simulink model "all_sliding_mode_z_trajectory_extension_v1"  (R2016b)
settings: Solver=ode4  StartTime=0.0  StopTime=t_stop  FixedStep=t_step  MaxStep=0.00001  MinStep=0.00000000001  RelTol=1e-3  EnableMultiTasking=on
values from neighbouring files (symbols this model uses):
  g = single(9.81)    [covert_pressure_to_height.m]
undefined symbols (not defined in the file or in its folder): a1, a2, a3, a4, a5, a6, b, cm, ct, d, disturbance, fd, Ix, Ixx, Iy, Iyy, Iz, Izz, k1, k2, k3, k4, k5, k6, Kd_phi, Kd_theta, Kd_x, Kd_y, Kd_z, Ki_phi, Ki_theta, Ki_x, Ki_y, Ki_z, Kp_phi, Kp_theta, Kp_x, Kp_y, Kp_z, L, l1, l2, l3, l4, l5, l6, m, O, phi_init, phi_ref, psi_init, psi_ref, smc, tau_att, tau_att_1, tau_p, theta_init, theta_ref, xref, yref ... (+2)
libraries: simulink x2
settings Model: Creator=Ajinkya  LastModifiedBy=Ajinkya
settings SolverCC: ZeroCrossAlgorithm=Adaptive  AlgebraicLoopSolver=LineSearch
settings DataIOCC: LimitDataPoints=on  SaveFormat=StructureWithTime
settings OptimizationCC: DefaultParameterBehavior=Inlined  EfficientMapNaN2IntZero=off
settings DebuggingCC: ParameterOverflowMsg=warning  ParameterTunabilityLossMsg=error  SFUnexpectedBacktrackingDiag=warning  SFNoUnconditionalDefaultTransitionDiag=warning  SFExecutionAtInitializationDiag=none
settings HardwareCC: ProdBitPerSizeT=32  ProdBitPerPtrDiffT=32  ProdWordSize=32  ProdHWDeviceType=Specified  TargetBitPerPointer=64  TargetBitPerSizeT=64  TargetBitPerPtrDiffT=64  TargetLongLongMode=on  TargetIntDivRoundTo=Zero  TargetEndianess=LittleEndian  TargetWordSize=64  TargetHWDeviceType=MATLAB Host  ProdEqTarget=off
settings ModelReferenceCC: PropagateSignalLabelsOutOfModel=off
settings RTWCC: GenerateReport=on  LaunchReport=on
settings CodeAppCC: ForceParamTrailComments=on  MaxIdLength=128  OperatorAnnotations=on  MATLABSourceComments=on
settings GRTTargetCC: TargetLangStandard=C89/C90 (ANSI)
settings ConfigComp: CovMetricSettings=dw  CovHtmlReporting=on  CovSaveCumulativeToWorkspaceVar=on  CovSaveSingleToWorkspaceVar=on  CovExternalEMLEnable=off

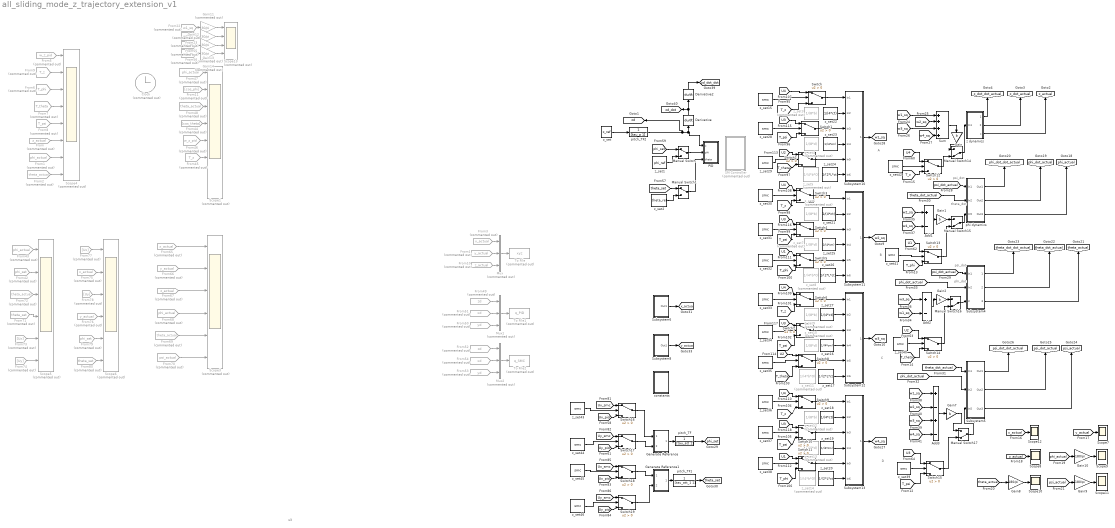
== system all_sliding_mode_z_trajectory_extension_v1 ==
  note: s3
  note: theta_dot
  note: psi_dot
  note: phi_dot
  note: psi_dot
  note: D
  note: C
  note: B
  note: A
  Add1 : Sum  Inputs=+-
  Add2 : Sum  Inputs=+-
  Add3 : Sum  Inputs=+-+-
  Clock : Clock  Commented=on
  Derivative : Derivative
  Derivative2 : Derivative
  From : From  Commented=on  GotoTag=z_actual  TagVisibility=global
  From{1,43,47,68} (4 alike) : From  Commented=on  GotoTag=phi_actual  TagVisibility=global
  From10 : From  Commented=on  GotoTag=z_actual  TagVisibility=global
  From11 : From  Commented=on  GotoTag=cos_phi
  From{2,48,69,72} (4 alike) : From  Commented=on  GotoTag=theta_actual  TagVisibility=global
  From22 : From  Commented=on  GotoTag=w1_sq  TagVisibility=global
  From23 : From  Commented=on  GotoTag=w2_sq  TagVisibility=global
  From3 : From  Commented=on  GotoTag=x_actual  TagVisibility=global
  From4 : From  Commented=on  GotoTag=y_actual  TagVisibility=global
  From42 : From  Commented=on  GotoTag=phi_set  TagVisibility=global
  From44 : From  Commented=on  GotoTag=cos_theta
  From45 : From  Commented=on  GotoTag=T_z  TagVisibility=global
  From46 : From  Commented=on  GotoTag=w_z_pid  TagVisibility=global
  From49 : From  Commented=on  GotoTag=zd  TagVisibility=global
  From5 : From  Commented=on  GotoTag=w_z_pid
  From50 : From  Commented=on  GotoTag=yd  TagVisibility=global
  From51 : From  Commented=on  GotoTag=xd  TagVisibility=global
  From52 : From  Commented=on  GotoTag=zd
  From53 : From  Commented=on  GotoTag=yd
  From54 : From  Commented=on  GotoTag=xd
  From55 : From  Commented=on  GotoTag=w3_sq  TagVisibility=global
  From56 : From  Commented=on  GotoTag=w4_sq  TagVisibility=global
  From6 : From  Commented=on  GotoTag=T_phi
  From65 : From  Commented=on  GotoTag=x_actual  TagVisibility=global
  From66 : From  Commented=on  GotoTag=y_actual  TagVisibility=global
  From67 : From  Commented=on  GotoTag=z_actual  TagVisibility=global
  From7 : From  Commented=on  GotoTag=T_theta
  From70 : From  Commented=on  GotoTag=psi_actual  TagVisibility=global
  From71 : From  Commented=on  GotoTag=theta_set  TagVisibility=global
  From73 : From  Commented=on  GotoTag=Ux
  From74 : From  Commented=on  GotoTag=Uy
  From75 : From  Commented=on  GotoTag=x_actual  TagVisibility=global
  From76 : From  Commented=on  GotoTag=y_actual  TagVisibility=global
  From77 : From  Commented=on  GotoTag=Ux
  From78 : From  Commented=on  GotoTag=Uy
  From79 : From  Commented=on  GotoTag=phi_set  TagVisibility=global
  From8 : From  Commented=on  GotoTag=T_psi
  From80 : From  Commented=on  GotoTag=theta_set  TagVisibility=global
  From9 : From  Commented=on  GotoTag=T_z
  Gain{,1..2,7} (4 alike) : Gain  Gain=b
  Gain10 : Gain  Gain=180/pi
  Gain{11..14} (4 alike) : Gain  Commented=on  Gain=30/pi
  Gain8 : Gain  Gain=180/pi
  Gain9 : Gain  Gain=180/pi
  Generate Reference : Subsystem
  Generate Reference1 : Subsystem
  Manual Switch : ManualSwitch
  Manual Switch1 : ManualSwitch
  Manual Switch{14..17} (4 alike) : ManualSwitch  CurrentSetting=0
  Mux : Mux  Commented=on  Inputs=3
  Mux1 : Mux  Commented=on  Inputs=3
  Mux2 : Mux  Commented=on  Inputs=3
  PID : Subsystem
  SM Controller : Subsystem  Commented=on
  Scope1 : Scope  Commented=on  NumInputPorts=8
  Scope{7..12} (6 alike) : Scope
  Scope13 : Scope  Commented=on  NumInputPorts=4
  Scope3 : Scope  Commented=on  NumInputPorts=6
  Scope4 : Scope  Commented=on  NumInputPorts=8
  Scope5 : Scope  Commented=on  NumInputPorts=6
  Scope6 : Scope  Commented=on  NumInputPorts=6
  Subsystem10 : Subsystem
  Subsystem11 : Subsystem
  Subsystem12 : Subsystem
  Subsystem13 : Subsystem
  Subsystem4 : Subsystem
  Subsystem5 : Subsystem
  Subsystem6 : Subsystem
  Subsystem8 : Subsystem
  Sum : Sum  Inputs=++++
  Switch{,1..19} (20 alike) : Switch  Criteria=u2 > Threshold
  To File : ToFile  Commented=on  Filename=xyz  MatrixName=xyz
  To File1 : ToFile  Commented=on  Filename=q_PID  MatrixName=q_PID
  To File2 : ToFile  Commented=on  Filename=q_SMC  MatrixName=q_SMC
  constants : Subsystem
  phi dynamics : Subsystem
  pitch_TF : TransferFcn  Denominator=[tau_att 1]
  pitch_TF1 : TransferFcn  Denominator=[tau_att_1 1]
  pitch_TF2 : TransferFcn  Denominator=[tau_p 1]
  z dynamics : Subsystem
  z_set : Constant  Value=z_ref
  z_set1 : Constant  Value=phi_ref
  z_set{4,7,10,13} (4 alike) : Constant  Commented=on  Value=1/(8*d)
  z_set{5,8,11,14} (4 alike) : Constant  Commented=on  Value=1/(4*b*O)
  z_set{3,6,9,12} (4 alike) : Constant  Commented=on  Value=1/(8*b)
  z_set{15,28..46} (20 alike) : Constant  Value=smc
  z_set{16,19,23,25} (4 alike) : Constant  Value=1/(4*cm)
  z_set{17,20,24,26} (4 alike) : Constant  Value=1/(2*L*ct)
  z_set{18,21..22,27} (4 alike) : Constant  Value=1/(4*ct)
  z_set2 : Constant  Value=theta_ref
  tag scope: phi_actual=global, phi_dot_actual=global, phi_dot_dot_actual=global, phi_set=global, psi_actual=global, psi_dot_actual=global, psi_dot_dot_actual=global, theta_actual=global, theta_dot_actual=global, theta_dot_dot_actual=global, theta_set=global, w1_sq=global, w2_sq=global, w3_sq=global, w4_sq=global, x_actual=global, y_actual=global, z_actual=global, z_dot_actual=global, z_dot_dot_actual=global, zd=global, zd_dot=global, zd_dot_dot=global
  wires:
  z_set/1 -> pitch_TF2/1
  z dynamics/1(z dot dot) -> [z_dot_dot_actual]
  z dynamics/2(z dot) -> [z_dot_actual]
  z dynamics/3(z) -> [z_actual]
  [w1_sq] -> Sum/1
  [w2_sq] -> Sum/2
  [w3_sq] -> Sum/3
  [w4_sq] -> Sum/4
  [psi_dot_actual] -> phi dynamics/1(In1)
  [theta_dot_actual] -> phi dynamics/2(In2)
  phi dynamics/1(Out1) -> [phi_dot_dot_actual]
  phi dynamics/2(Out2) -> [phi_dot_actual]
  phi dynamics/3(Out3) -> [phi_actual]
  [psi_dot_actual] -> Subsystem4/1(In1)
  [phi_dot_actual] -> Subsystem4/2(In2)
  Subsystem4/1(Out1) -> [theta_dot_dot_actual]
  Subsystem4/2(Out2) -> [theta_dot_actual]
  Subsystem4/3(Out3) -> [theta_actual]
  [theta_dot_actual] -> Subsystem5/1(In1)
  [phi_dot_actual] -> Subsystem5/2(In2)
  Subsystem5/1(Out1) -> [psi_dot_dot_actual]
  Subsystem5/2(Out2) -> [psi_dot_actual]
  Subsystem5/3(Out3) -> [psi_actual]
  From2/1 -> Scope4/8
  From1/1 -> Scope4/7
  From/1 -> Scope4/6
  From8/1 -> Scope4/5
  From7/1 -> Scope4/4
  From6/1 -> Scope4/3
  From9/1 -> Scope4/2
  From5/1 -> Scope4/1
  From11/1 -> Scope1/2
  From44/1 -> Scope1/4
  From45/1 -> Scope1/6
  From46/1 -> Scope1/5
  From48/1 -> Scope1/3
  From47/1 -> Scope1/1
  [w1_sq] -> Add2/2
  [w4_sq] -> Add3/4
  [w3_sq] -> Add3/3
  [w2_sq] -> Add3/2
  z_set1/1 -> Manual Switch/2
  [phi_set] -> Manual Switch/1
  z_set2/1 -> Manual Switch1/2
  [theta_set] -> Manual Switch1/1
  Subsystem6/1(Out1) -> [x_actual]
  Subsystem8/1(Out1) -> [y_actual]
  From65/1 -> Scope3/1
  From66/1 -> Scope3/2
  From67/1 -> Scope3/3
  From68/1 -> Scope3/4
  From69/1 -> Scope3/5
  From70/1 -> Scope3/6
  From42/1 -> Scope5/2
  From43/1 -> Scope5/1
  From71/1 -> Scope5/4
  From72/1 -> Scope5/3
  From73/1 -> Scope5/5
  From74/1 -> Scope5/6
  From75/1 -> Scope6/2
  From76/1 -> Scope6/4
  From77/1 -> Scope6/1
  From78/1 -> Scope6/3
  From79/1 -> Scope6/5
  From80/1 -> Scope6/6
  Derivative/1 -> [zd_dot], Derivative2/1
  Derivative2/1 -> [zd_dot_dot]
  Sum/1 -> Gain/1
  Manual Switch14/1 -> z dynamics/1(In1)
  Gain/1 -> Manual Switch14/1
  [w2_sq] -> Add1/1
  [w4_sq] -> Add1/2
  Manual Switch15/1 -> phi dynamics/3(In5)
  [w3_sq] -> Add2/1
  Manual Switch16/1 -> Subsystem4/3(w3_sq)
  Add1/1 -> Gain1/1
  Gain1/1 -> Manual Switch15/1
  Gain2/1 -> Manual Switch16/1
  Add2/1 -> Gain2/1
  [w1_sq] -> Add3/1
  Add3/1 -> Gain7/1
  Gain7/1 -> Manual Switch17/1
  Manual Switch17/1 -> Subsystem5/3(In5)
  z_set22/1 -> Subsystem10/2(In2)
  z_set23/1 -> Subsystem10/4(In4)
  z_set24/1 -> Subsystem10/6(In6)
  z_set21/1 -> Subsystem11/2(In2)
  z_set25/1 -> Subsystem11/4(In4)
  z_set26/1 -> Subsystem11/6(In6)
  z_set27/1 -> Subsystem12/2(In2)
  z_set16/1 -> Subsystem12/4(In4)
  z_set17/1 -> Subsystem12/6(In6)
  z_set18/1 -> Subsystem13/2(In2)
  z_set19/1 -> Subsystem13/4(In4)
  z_set20/1 -> Subsystem13/6(In6)
  Subsystem10/1(w1_sq) -> [w1_sq]
  Subsystem11/1(w2_sq) -> [w2_sq]
  Subsystem12/1(w3_sq) -> [w3_sq]
  Subsystem13/1(w4_sq) -> [w4_sq]
  [T_z] -> Switch/3
  Switch/1 -> Subsystem10/1(In1)
  [U4] -> Switch/1
  [T_z] -> Switch3/3
  [U4] -> Switch3/1
  Switch3/1 -> Subsystem11/1(In1)
  [T_z] -> Switch6/3
  Switch6/1 -> Subsystem12/1(In1)
  [U4] -> Switch6/1
  [T_z] -> Switch9/3
  Switch9/1 -> Subsystem13/1(In1)
  [U4] -> Switch9/1
  Switch1/1 -> Subsystem10/3(In3)
  [T_psi] -> Switch1/3
  Switch2/1 -> Subsystem10/5(In5)
  [T_theta] -> Switch2/3
  [T_psi] -> Switch4/3
  Switch4/1 -> Subsystem11/3(In3)
  Switch5/1 -> Subsystem11/5(In5)
  [T_phi] -> Switch5/3
  Switch7/1 -> Subsystem12/3(In3)
  [T_psi] -> Switch7/3
  Switch8/1 -> Subsystem12/5(In5)
  [T_theta] -> Switch8/3
  Switch10/1 -> Subsystem13/3(In3)
  [T_psi] -> Switch10/3
  Switch11/1 -> Subsystem13/5(In5)
  [T_phi] -> Switch11/3
  [U1] -> Switch5/1
  [U1] -> Switch11/1
  [U2] -> Switch2/1
  [U2] -> Switch8/1
  [U3] -> Switch1/1
  [U3] -> Switch4/1
  [U3] -> Switch7/1
  [U3] -> Switch10/1
  Switch12/1 -> Manual Switch14/2
  [U1] -> Switch13/1
  Switch13/1 -> Manual Switch15/2
  [U2] -> Switch14/1
  Switch14/1 -> Manual Switch16/2
  [U3] -> Switch15/1
  Switch15/1 -> Manual Switch17/2
  [T_psi] -> Switch15/3
  [T_phi] -> Switch13/3
  [T_theta] -> Switch14/3
  Manual Switch/1 -> PID/2(phi)
  Manual Switch1/1 -> PID/3(theta)
  [x_actual] -> Scope12/1
  [z_actual] -> Scope8/1
  [y_actual] -> Scope7/1
  Generate Reference/1(Out1) -> pitch_TF/1
  pitch_TF/1 -> [phi_set]
  Generate Reference1/1(Out1) -> pitch_TF1/1
  [psi_actual] -> Gain9/1
  [phi_actual] -> Gain10/1
  From22/1 -> Gain11/1
  Gain11/1 -> Scope13/1
  Gain12/1 -> Scope13/2
  From23/1 -> Gain12/1
  From55/1 -> Gain13/1
  Gain13/1 -> Scope13/3
  From56/1 -> Gain14/1
  Gain14/1 -> Scope13/4
  Gain9/1 -> Scope11/1
  Gain8/1 -> Scope10/1
  Gain10/1 -> Scope9/1
  [theta_actual] -> Gain8/1
  z_set15/1 -> Switch/2
  z_set28/1 -> Switch1/2
  z_set29/1 -> Switch2/2
  z_set30/1 -> Switch3/2
  z_set31/1 -> Switch4/2
  z_set32/1 -> Switch5/2
  z_set33/1 -> Switch6/2
  z_set34/1 -> Switch7/2
  z_set35/1 -> Switch8/2
  z_set36/1 -> Switch9/2
  z_set37/1 -> Switch10/2
  z_set38/1 -> Switch11/2
  [T_z] -> Switch12/3
  [U4] -> Switch12/1
  z_set39/1 -> Switch15/2
  z_set40/1 -> Switch14/2
  z_set41/1 -> Switch13/2
  z_set42/1 -> Switch12/2
  Mux/1 -> To File/1
  From3/1 -> Mux/1
  From4/1 -> Mux/2
  From10/1 -> Mux/3
  From50/1 -> Mux1/3
  From51/1 -> Mux1/2
  From49/1 -> Mux1/1
  Mux1/1 -> To File1/1
  From53/1 -> Mux2/3
  From54/1 -> Mux2/2
  From52/1 -> Mux2/1
  Mux2/1 -> To File2/1
  pitch_TF2/1 -> [zd], PID/1(z), Derivative/1
  pitch_TF1/1 -> [theta_set]
  [Ux_smc] -> Switch16/1
  [Ux_pid] -> Switch16/3
  [Uy_smc] -> Switch17/1
  [Uy_pid] -> Switch17/3
  z_set43/1 -> Switch16/2
  z_set44/1 -> Switch17/2
  Switch16/1 -> Generate Reference/1(In1)
  Switch17/1 -> Generate Reference/2(In2)
  [Ux_smc] -> Switch18/1
  [Ux_pid] -> Switch18/3
  [Uy_smc] -> Switch19/1
  [Uy_pid] -> Switch19/3
  z_set45/1 -> Switch18/2
  z_set46/1 -> Switch19/2
  Switch18/1 -> Generate Reference1/1(In1)
  Switch19/1 -> Generate Reference1/2(In2)

== system all_sliding_mode_z_trajectory_extension_v1/Generate Reference ==
  In1 : Inport
  In2 : Inport  Port=2
  Product1 : Product
  Product11 : Product
  Sum1 : Sum  Inputs=+-
  Trigonometric Function2 : Trigonometry  Operator=asin  OutputSignalType=real
  Trigonometric Function3 : Trigonometry
  Trigonometric Function4 : Trigonometry  Operator=cos
  Out1 : Outport
  wires:
  Product1/1 -> Sum1/2
  Product11/1 -> Sum1/1
  Trigonometric Function4/1 -> Product1/2
  Sum1/1 -> Trigonometric Function2/1
  Trigonometric Function2/1 -> Out1/1
  [psi_actual] -> Trigonometric Function4/1
  [psi_actual] -> Trigonometric Function3/1
  Trigonometric Function3/1 -> Product11/1
  In1/1 -> Product11/2
  In2/1 -> Product1/1

== system all_sliding_mode_z_trajectory_extension_v1/Generate Reference1 ==
  In1 : Inport
  In2 : Inport  Port=2
  Divide : Product  Inputs=*/
  Product1 : Product
  Product11 : Product
  Sum1 : Sum
  Trigonometric Function1 : Trigonometry  Operator=cos
  Trigonometric Function2 : Trigonometry  Operator=asin  OutputSignalType=real
  Trigonometric Function3 : Trigonometry  Operator=cos
  Trigonometric Function4 : Trigonometry
  Out1 : Outport
  wires:
  Product1/1 -> Sum1/2
  Product11/1 -> Sum1/1
  Trigonometric Function4/1 -> Product1/2
  Trigonometric Function2/1 -> Out1/1
  [psi_actual] -> Trigonometric Function4/1
  [psi_actual] -> Trigonometric Function3/1
  Trigonometric Function3/1 -> Product11/1
  Sum1/1 -> Divide/1
  Divide/1 -> Trigonometric Function2/1
  [phi_set] -> Trigonometric Function1/1
  Trigonometric Function1/1 -> Divide/2
  In1/1 -> Product11/2
  In2/1 -> Product1/1

== system all_sliding_mode_z_trajectory_extension_v1/PID ==
  z : Inport
  phi : Inport  Port=2
  theta : Inport  Port=3
  Subsystem7 : Subsystem
  Subsystem9 : Subsystem
  T_phi : Subsystem
  T_psi : Subsystem
  T_theta : Subsystem
  T_z : Subsystem
  z_set3 : Constant  Value=psi_ref
  tag scope: T_phi=global, T_psi=global, T_theta=global, T_z=global, Ux_pid=global, Uy_pid=global
  wires:
  z/1 -> T_z/1(zref)
  phi/1 -> T_phi/1(phi ref)
  theta/1 -> T_theta/1(theta ref)
  T_z/1(Tz) -> [T_z]
  T_phi/1(T_phi) -> [T_phi]
  T_theta/1(T_theta) -> [T_theta]
  z_set3/1 -> T_psi/1(psi ref)
  T_psi/1(T_psi) -> [T_psi]
  [x_actual] -> Subsystem7/1(In1)
  Subsystem7/1(Out1) -> [Ux_pid]
  [y_actual] -> Subsystem9/1(In1)
  Subsystem9/1(Out1) -> [Uy_pid]

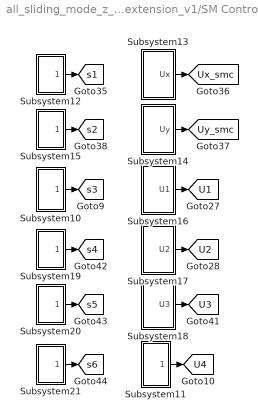
== system all_sliding_mode_z_trajectory_extension_v1/SM Controller ==
  Subsystem10 : Subsystem
  Subsystem11 : Subsystem
  Subsystem12 : Subsystem
  Subsystem13 : Subsystem
  Subsystem14 : Subsystem
  Subsystem15 : Subsystem
  Subsystem16 : Subsystem
  Subsystem17 : Subsystem
  Subsystem18 : Subsystem
  Subsystem19 : Subsystem
  Subsystem20 : Subsystem
  Subsystem21 : Subsystem
  tag scope: U1=global, U2=global, U3=global, U4=global, Ux_smc=global, Uy_smc=global, s1=global, s2=global, s3=global, s4=global, s5=global, s6=global
  wires:
  Subsystem19/1(s4) -> [s4]
  Subsystem17/1(U2) -> [U2]
  Subsystem18/1(U3) -> [U3]
  Subsystem16/1(U1) -> [U1]
  Subsystem12/1(s1) -> [s1]
  Subsystem15/1(s2) -> [s2]
  Subsystem10/1(s3) -> [s3]
  Subsystem11/1(U4) -> [U4]
  Subsystem13/1(Ux) -> [Ux_smc]
  Subsystem14/1(Uy) -> [Uy_smc]
  Subsystem20/1(s5) -> [s5]
  Subsystem21/1(s6) -> [s6]

== system all_sliding_mode_z_trajectory_extension_v1/Subsystem10 ==
  In1 : Inport
  In2 : Inport  Port=2
  In3 : Inport  Port=3
  In4 : Inport  Port=4
  In5 : Inport  Port=5
  In6 : Inport  Port=6
  Product1 : Product
  Product10 : Product
  Product9 : Product
  Saturation6 : Saturate  UpperLimit=11000*11000  LowerLimit=0
  Sum : Sum  Inputs=+--
  w1_sq : Outport
  wires:
  Product1/1 -> Sum/1
  Product9/1 -> Sum/2
  Sum/1 -> Saturation6/1
  Product10/1 -> Sum/3
  In1/1 -> Product1/1
  In2/1 -> Product1/2
  In4/1 -> Product9/2
  In5/1 -> Product10/1
  In3/1 -> Product9/1
  In6/1 -> Product10/2
  Saturation6/1 -> w1_sq/1

== system all_sliding_mode_z_trajectory_extension_v1/Subsystem11 ==
  In1 : Inport
  In2 : Inport  Port=2
  In3 : Inport  Port=3
  In4 : Inport  Port=4
  In5 : Inport  Port=5
  In6 : Inport  Port=6
  Product1 : Product
  Product10 : Product
  Product9 : Product
  Saturation6 : Saturate  UpperLimit=11000*11000  LowerLimit=0
  Sum : Sum  Inputs=++-
  w2_sq : Outport
  wires:
  Product1/1 -> Sum/1
  Product9/1 -> Sum/2
  Sum/1 -> Saturation6/1
  Product10/1 -> Sum/3
  In1/1 -> Product1/1
  In2/1 -> Product1/2
  In4/1 -> Product9/2
  In5/1 -> Product10/1
  In3/1 -> Product9/1
  In6/1 -> Product10/2
  Saturation6/1 -> w2_sq/1

== system all_sliding_mode_z_trajectory_extension_v1/Subsystem12 ==
  In1 : Inport
  In2 : Inport  Port=2
  In3 : Inport  Port=3
  In4 : Inport  Port=4
  In5 : Inport  Port=5
  In6 : Inport  Port=6
  Product1 : Product
  Product10 : Product
  Product9 : Product
  Saturation6 : Saturate  UpperLimit=11000*11000  LowerLimit=0
  Sum : Sum  Inputs=+-+
  w3_sq : Outport
  wires:
  Product1/1 -> Sum/1
  Product9/1 -> Sum/2
  Sum/1 -> Saturation6/1
  Product10/1 -> Sum/3
  In1/1 -> Product1/1
  In2/1 -> Product1/2
  In4/1 -> Product9/2
  In5/1 -> Product10/1
  In3/1 -> Product9/1
  In6/1 -> Product10/2
  Saturation6/1 -> w3_sq/1

== system all_sliding_mode_z_trajectory_extension_v1/Subsystem13 ==
  In1 : Inport
  In2 : Inport  Port=2
  In3 : Inport  Port=3
  In4 : Inport  Port=4
  In5 : Inport  Port=5
  In6 : Inport  Port=6
  Product1 : Product
  Product10 : Product
  Product9 : Product
  Saturation6 : Saturate  UpperLimit=11000*11000  LowerLimit=0
  Sum : Sum  Inputs=+++
  w4_sq : Outport
  wires:
  Product1/1 -> Sum/1
  Product9/1 -> Sum/2
  Sum/1 -> Saturation6/1
  Product10/1 -> Sum/3
  In1/1 -> Product1/1
  In2/1 -> Product1/2
  In4/1 -> Product9/2
  In5/1 -> Product10/1
  In3/1 -> Product9/1
  In6/1 -> Product10/2
  Saturation6/1 -> w4_sq/1

== system all_sliding_mode_z_trajectory_extension_v1/Subsystem4 ==
  note: theta
  note: theta_dot
  note: theta_dot_dot
  In1 : Inport
  In2 : Inport  Port=2
  w3_sq : Inport  Port=3
  Integrator4 : Integrator
  Integrator5 : Integrator  InitialCondition=theta_init
  Product4 : Product  Inputs=3
  Product5 : Product
  Scope1 : Scope  NumInputPorts=5
  Subtract2 : Sum
  b/m3 : Constant  Value=(-Izz+Ixx)/Iyy
  b/m4 : Constant  Value=1/Iyy
  Out1 : Outport
  Out2 : Outport  Port=2
  Out3 : Outport  Port=3
  wires:
  In1/1 -> Product4/2
  In2/1 -> Product4/3
  Product4/1 -> Scope1/1, Subtract2/1
  b/m3/1 -> Product4/1
  b/m4/1 -> Product5/1
  Product5/1 -> Subtract2/2
  Integrator4/1 -> Out2/1, Scope1/4, Integrator5/1
  w3_sq/1 -> Scope1/2, Product5/2
  Integrator5/1 -> Scope1/5, Out3/1
  Subtract2/1 -> Scope1/3, Out1/1, Integrator4/1

== system all_sliding_mode_z_trajectory_extension_v1/Subsystem5 ==
  note: psi
  note: psi_dot
  note: psi_dot_dot
  note: phi_dot
  note: theta_dot
  In1 : Inport
  In2 : Inport  Port=2
  In5 : Inport  Port=3
  Integrator6 : Integrator
  Integrator7 : Integrator  InitialCondition=psi_init
  Product6 : Product  Inputs=3
  Product7 : Product
  Scope3 : Scope  NumInputPorts=3
  Subtract3 : Sum
  b/m5 : Constant  Value=(Ixx-Iyy)/Izz
  b/m6 : Constant  Value=1/Izz
  Out1 : Outport
  Out2 : Outport  Port=2
  Out3 : Outport  Port=3
  wires:
  Integrator7/1 -> Out3/1, Scope3/1
  In2/1 -> Product6/3
  b/m5/1 -> Product6/1
  b/m6/1 -> Product7/1
  Subtract3/1 -> Out1/1, Integrator6/1
  Product7/1 -> Subtract3/2
  Product6/1 -> Subtract3/1
  Integrator6/1 -> Out2/1, Integrator7/1
  In5/1 -> Product7/2
  In1/1 -> Product6/2

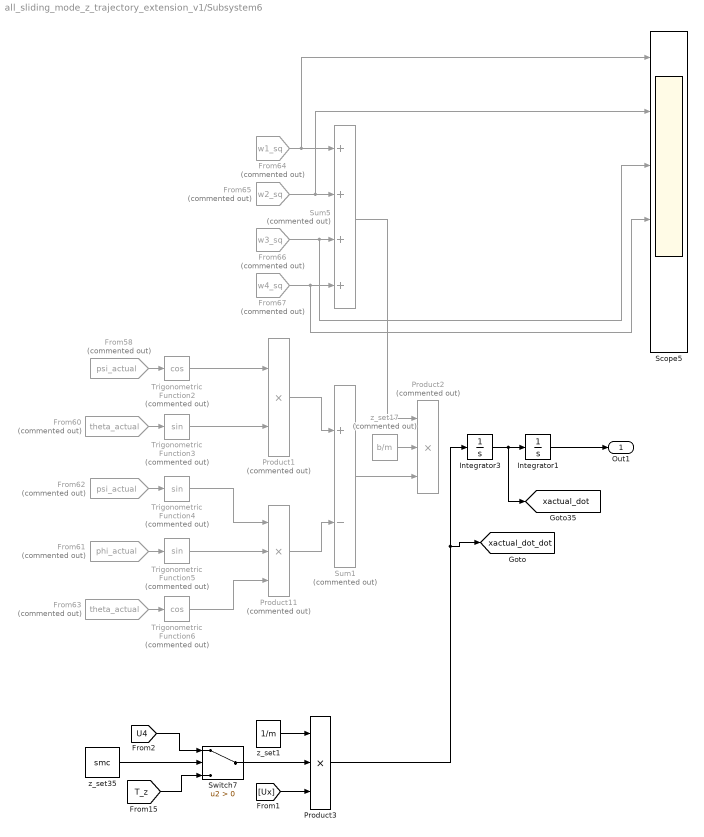
== system all_sliding_mode_z_trajectory_extension_v1/Subsystem6 ==
  From58 : From  Commented=on  GotoTag=psi_actual  TagVisibility=global
  From60 : From  Commented=on  GotoTag=theta_actual  TagVisibility=global
  From61 : From  Commented=on  GotoTag=phi_actual  TagVisibility=global
  From62 : From  Commented=on  GotoTag=psi_actual  TagVisibility=global
  From63 : From  Commented=on  GotoTag=theta_actual  TagVisibility=global
  From64 : From  Commented=on  GotoTag=w1_sq  TagVisibility=global
  From65 : From  Commented=on  GotoTag=w2_sq  TagVisibility=global
  From66 : From  Commented=on  GotoTag=w3_sq  TagVisibility=global
  From67 : From  Commented=on  GotoTag=w4_sq  TagVisibility=global
  Integrator1 : Integrator  InitialCondition=phi_init
  Integrator3 : Integrator  InitialCondition=phi_init
  Product1 : Product  Commented=on
  Product11 : Product  Commented=on  Inputs=3
  Product2 : Product  Commented=on  Inputs=3
  Product3 : Product  Inputs=3
  Scope5 : Scope  NumInputPorts=6
  Sum1 : Sum  Commented=on  Inputs=+-
  Sum5 : Sum  Commented=on  Inputs=++++
  Switch7 : Switch  Criteria=u2 > Threshold
  Trigonometric Function2 : Trigonometry  Commented=on  Operator=cos
  Trigonometric Function3 : Trigonometry  Commented=on
  Trigonometric Function4 : Trigonometry  Commented=on
  Trigonometric Function5 : Trigonometry  Commented=on
  Trigonometric Function6 : Trigonometry  Commented=on  Operator=cos
  z_set1 : Constant  Value=1/m
  z_set17 : Constant  Commented=on  Value=b/m
  z_set35 : Constant  Value=smc
  Out1 : Outport
  tag scope: xactual_dot=global, xactual_dot_dot=global
  wires:
  Trigonometric Function3/1 -> Product1/2
  From60/1 -> Trigonometric Function3/1
  From61/1 -> Trigonometric Function5/1
  From58/1 -> Trigonometric Function2/1
  Trigonometric Function5/1 -> Product11/2
  Trigonometric Function6/1 -> Product11/3
  Trigonometric Function4/1 -> Product11/1
  From62/1 -> Trigonometric Function4/1
  Trigonometric Function2/1 -> Product1/1
  From63/1 -> Trigonometric Function6/1
  z_set17/1 -> Product2/2
  From67/1 -> Scope5/4, Sum5/4
  Sum5/1 -> Product2/1
  Product1/1 -> Sum1/1
  Product11/1 -> Sum1/2
  Integrator3/1 -> [xactual_dot], Integrator1/1
  Integrator1/1 -> Out1/1
  From64/1 -> Sum5/1, Scope5/1
  From66/1 -> Scope5/3, Sum5/3
  From65/1 -> Scope5/2, Sum5/2
  Sum1/1 -> Product2/3
  Switch7/1 -> Product3/2
  z_set1/1 -> Product3/1
  Product3/1 -> [xactual_dot_dot], Integrator3/1
  [Ux] -> Product3/3
  [U4] -> Switch7/1
  [T_z] -> Switch7/3
  z_set35/1 -> Switch7/2

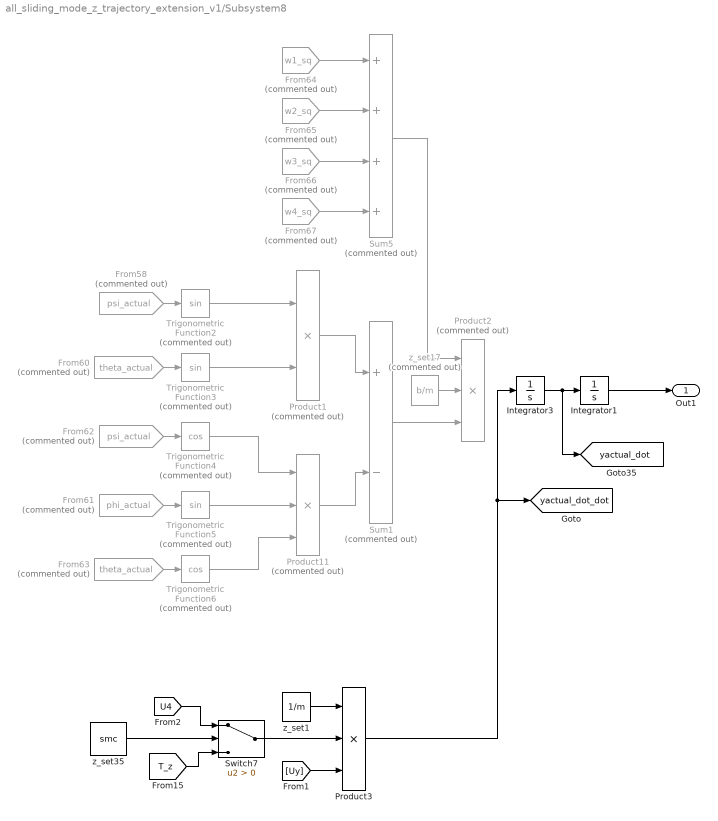
== system all_sliding_mode_z_trajectory_extension_v1/Subsystem8 ==
  From58 : From  Commented=on  GotoTag=psi_actual  TagVisibility=global
  From60 : From  Commented=on  GotoTag=theta_actual  TagVisibility=global
  From61 : From  Commented=on  GotoTag=phi_actual  TagVisibility=global
  From62 : From  Commented=on  GotoTag=psi_actual  TagVisibility=global
  From63 : From  Commented=on  GotoTag=theta_actual  TagVisibility=global
  From64 : From  Commented=on  GotoTag=w1_sq  TagVisibility=global
  From65 : From  Commented=on  GotoTag=w2_sq  TagVisibility=global
  From66 : From  Commented=on  GotoTag=w3_sq  TagVisibility=global
  From67 : From  Commented=on  GotoTag=w4_sq  TagVisibility=global
  Integrator1 : Integrator  InitialCondition=phi_init
  Integrator3 : Integrator  InitialCondition=phi_init
  Product1 : Product  Commented=on
  Product11 : Product  Commented=on  Inputs=3
  Product2 : Product  Commented=on  Inputs=3
  Product3 : Product  Inputs=3
  Sum1 : Sum  Commented=on  Inputs=+-
  Sum5 : Sum  Commented=on  Inputs=++++
  Switch7 : Switch  Criteria=u2 > Threshold
  Trigonometric Function2 : Trigonometry  Commented=on
  Trigonometric Function3 : Trigonometry  Commented=on
  Trigonometric Function4 : Trigonometry  Commented=on  Operator=cos
  Trigonometric Function5 : Trigonometry  Commented=on
  Trigonometric Function6 : Trigonometry  Commented=on  Operator=cos
  z_set1 : Constant  Value=1/m
  z_set17 : Constant  Commented=on  Value=b/m
  z_set35 : Constant  Value=smc
  Out1 : Outport
  tag scope: yactual_dot=global, yactual_dot_dot=global
  wires:
  Trigonometric Function3/1 -> Product1/2
  From60/1 -> Trigonometric Function3/1
  From61/1 -> Trigonometric Function5/1
  From58/1 -> Trigonometric Function2/1
  Trigonometric Function5/1 -> Product11/2
  Trigonometric Function6/1 -> Product11/3
  Trigonometric Function4/1 -> Product11/1
  From62/1 -> Trigonometric Function4/1
  Trigonometric Function2/1 -> Product1/1
  From63/1 -> Trigonometric Function6/1
  z_set17/1 -> Product2/2
  From67/1 -> Sum5/4
  Sum5/1 -> Product2/1
  Product1/1 -> Sum1/1
  Product11/1 -> Sum1/2
  Integrator3/1 -> [yactual_dot], Integrator1/1
  Integrator1/1 -> Out1/1
  From64/1 -> Sum5/1
  From66/1 -> Sum5/3
  From65/1 -> Sum5/2
  Sum1/1 -> Product2/3
  Switch7/1 -> Product3/2
  z_set1/1 -> Product3/1
  Product3/1 -> [yactual_dot_dot], Integrator3/1
  [Uy] -> Product3/3
  [U4] -> Switch7/1
  [T_z] -> Switch7/3
  z_set35/1 -> Switch7/2

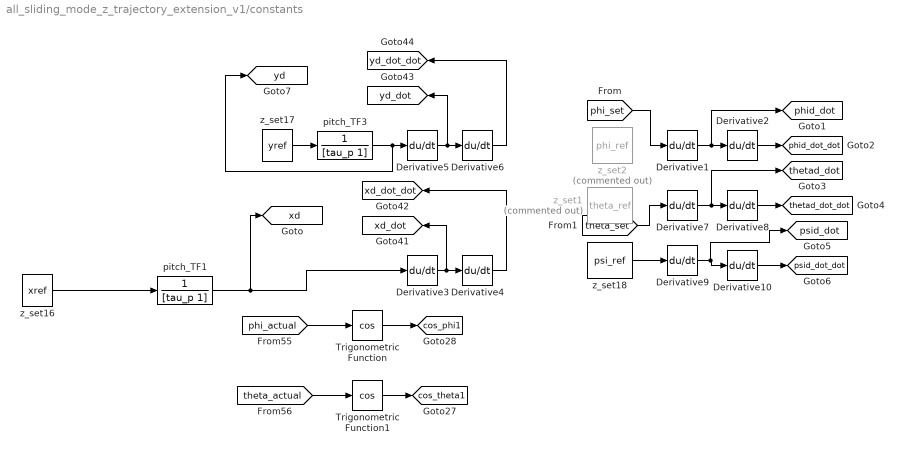
== system all_sliding_mode_z_trajectory_extension_v1/constants ==
  Derivative{1..10} (10 alike) : Derivative
  Trigonometric Function : Trigonometry  Operator=cos
  Trigonometric Function1 : Trigonometry  Operator=cos
  pitch_TF1 : TransferFcn  Denominator=[tau_p 1]
  pitch_TF3 : TransferFcn  Denominator=[tau_p 1]
  z_set1 : Constant  Commented=on  Value=theta_ref
  z_set16 : Constant  Value=xref
  z_set17 : Constant  Value=yref
  z_set18 : Constant  Value=psi_ref
  z_set2 : Constant  Commented=on  Value=phi_ref
  tag scope: cos_phi1=global, cos_theta1=global, phid_dot=global, phid_dot_dot=global, psid_dot=global, psid_dot_dot=global, thetad_dot=global, thetad_dot_dot=global, xd=global, xd_dot=global, xd_dot_dot=global, yd=global, yd_dot=global, yd_dot_dot=global
  wires:
  Derivative4/1 -> [xd_dot_dot]
  [theta_actual] -> Trigonometric Function1/1
  [phi_actual] -> Trigonometric Function/1
  Trigonometric Function/1 -> [cos_phi1]
  Trigonometric Function1/1 -> [cos_theta1]
  Derivative3/1 -> [xd_dot], Derivative4/1
  z_set16/1 -> pitch_TF1/1
  Derivative5/1 -> [yd_dot], Derivative6/1
  Derivative6/1 -> [yd_dot_dot]
  z_set17/1 -> pitch_TF3/1
  Derivative1/1 -> [phid_dot], Derivative2/1
  Derivative7/1 -> [thetad_dot], Derivative8/1
  z_set18/1 -> Derivative9/1
  Derivative9/1 -> [psid_dot], Derivative10/1
  Derivative2/1 -> [phid_dot_dot]
  Derivative8/1 -> [thetad_dot_dot]
  Derivative10/1 -> [psid_dot_dot]
  [theta_set] -> Derivative7/1
  [phi_set] -> Derivative1/1
  pitch_TF1/1 -> [xd], Derivative3/1
  pitch_TF3/1 -> [yd], Derivative5/1

== system all_sliding_mode_z_trajectory_extension_v1/phi dynamics ==
  note: phi
  note: phi_dot
  note: phi_dot_dot
  In1 : Inport
  In2 : Inport  Port=2
  In5 : Inport  Port=3
  Integrator2 : Integrator
  Integrator3 : Integrator  InitialCondition=phi_init
  Product2 : Product  Inputs=3
  Product3 : Product
  Scope1 : Scope  NumInputPorts=3
  Subtract1 : Sum
  b/m1 : Constant  Value=(Iyy-Izz)/Ixx
  b/m2 : Constant  Value=1/Ixx
  Out1 : Outport
  Out2 : Outport  Port=2
  Out3 : Outport  Port=3
  wires:
  In1/1 -> Product2/2
  b/m2/1 -> Product3/1
  In5/1 -> Product3/2
  Product3/1 -> Subtract1/2
  Integrator3/1 -> Out3/1, Scope1/1
  b/m1/1 -> Product2/1
  Subtract1/1 -> Out1/1, Integrator2/1
  Product2/1 -> Subtract1/1
  Integrator2/1 -> Out2/1, Integrator3/1
  In2/1 -> Product2/3

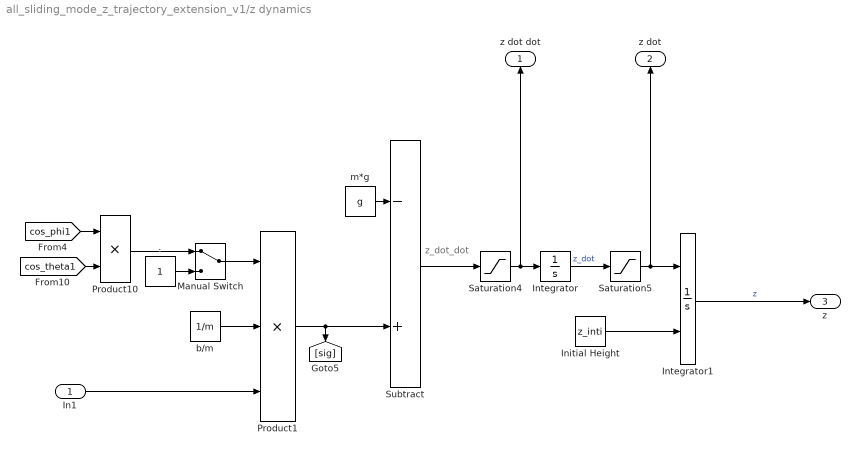
== system all_sliding_mode_z_trajectory_extension_v1/z dynamics ==
  note: z_dot_dot
  In1 : Inport
  . : Constant
  Initial Height : Constant  Value=z_inti
  Integrator : Integrator
  Integrator1 : Integrator  InitialConditionSource=external
  Manual Switch : ManualSwitch
  Product1 : Product  Inputs=3
  Product10 : Product
  Saturation4 : Saturate  UpperLimit=20  LowerLimit=-20
  Saturation5 : Saturate  UpperLimit=5  LowerLimit=-5
  Subtract : Sum  Inputs=-+
  b/m : Constant  Value=1/m
  m*g : Constant  Value=g
  z dot dot : Outport
  z dot : Outport  Port=2
  z : Outport  Port=3
  wires:
  Product10/1 -> Manual Switch/1
  m*g/1 -> Subtract/1
  b/m/1 -> Product1/2
  Integrator1/1 -> z/1  "z"
  Integrator/1 -> Saturation5/1  "z_dot"
  Initial Height/1 -> Integrator1/2
  Product1/1 -> Subtract/2, [sig]
  Manual Switch/1 -> Product1/1
  Saturation4/1 -> z dot dot/1, Integrator/1
  Saturation5/1 -> z dot/1, Integrator1/1
  Subtract/1 -> Saturation4/1
  ./1 -> Manual Switch/2
  In1/1 -> Product1/3
  [cos_phi1] -> Product10/1
  [cos_theta1] -> Product10/2

== system all_sliding_mode_z_trajectory_extension_v1/PID/Subsystem7 ==
  In1 : Inport
  Constant : Constant  Commented=on  Value=m/b
  Derivative{,1..3} (4 alike) : Derivative  Commented=on
  Divide : Product  Commented=on  Inputs=**/
  From64 : From  Commented=on  GotoTag=w1_sq  TagVisibility=global
  From65 : From  Commented=on  GotoTag=w2_sq  TagVisibility=global
  From66 : From  Commented=on  GotoTag=w3_sq  TagVisibility=global
  From67 : From  Commented=on  GotoTag=w4_sq  TagVisibility=global
  Goto8 : Goto  Commented=on  GotoTag=xd  TagVisibility=global
  PID Controller : simulink/Continuous/PID Controller  Controller=PID  TimeDomain=Continuous-time  SampleTime=-1  IntegratorMethod=Forward Euler  FilterMethod=Forward Euler  Form=Parallel  UseFilter=on  ControllerParametersSource=internal  P=Kp_x  I=Ki_x  D=Kd_x  N=100  InitialConditionSource=internal  InitialConditionForIntegrator=0  InitialConditionForFilter=0  ExternalReset=none  LimitOutput=off  UpperSaturationLimit=inf  LowerSaturationLimit=-inf  LinearizeAsGain=on  AntiWindupMode=none  Kb=1  TrackingMode=off  Kt=1  PParamMin=[]  PParamMax=[]  IParamMin=[]  IParamMax=[]  DParamMin=[]  DParamMax=[]  NParamMin=[]  NParamMax=[]  KbParamMin=[]  KbParamMax=[]  KtParamMin=[]  KtParamMax=[]  POutMin=[]  POutMax=[]  IOutMin=[]  IOutMax=[]  DOutMin=[]  DOutMax=[]  NOutMin=[]  NOutMax=[]  KbOutMin=[]  KbOutMax=[]  KtOutMin=[]  KtOutMax=[]  IntegratorOutMin=[]  IntegratorOutMax=[]  FilterOutMin=[]  FilterOutMax=[]  SumOutMin=[]  SumOutMax=[]  SumI1OutMin=[]  SumI1OutMax=[]  SumI2OutMin=[]  SumI2OutMax=[]  SumI3OutMin=[]  SumI3OutMax=[]  SumDOutMin=[]  SumDOutMax=[]  SaturationOutMin=[]  SaturationOutMax=[]  IntegratorContinuousStateAttributes=''  IntegratorStateMustResolveToSignalObject=off  IntegratorRTWStateStorageClass=Auto  FilterContinuousStateAttributes=''  FilterStateMustResolveToSignalObject=off  FilterRTWStateStorageClass=Auto  DifferentiatorICPrevScaledInput=0  DifferentiatorOutMin=[]  DifferentiatorOutMax=[]
  Sum5 : Sum  Commented=on  Inputs=++++  OutMin=[0.0001]
  Sum7 : Sum  Inputs=-+|
  pitch_TF2 : TransferFcn  Commented=on  Denominator=[tau_p 1]
  Out1 : Outport
  wires:
  From65/1 -> Sum5/2
  From64/1 -> Sum5/1
  From67/1 -> Sum5/4
  Sum5/1 -> Divide/3
  From66/1 -> Sum5/3
  In1/1 -> Sum7/1
  Constant/1 -> Divide/2
  Derivative/1 -> Derivative2/1
  Sum7/1 -> PID Controller/1
  PID Controller/1 -> Out1/1, Derivative1/1
  Derivative1/1 -> Derivative3/1
  [xd] -> Sum7/2, pitch_TF2/1

== system all_sliding_mode_z_trajectory_extension_v1/PID/Subsystem9 ==
  In1 : Inport
  Constant : Constant  Commented=on  Value=m/b
  Derivative : Derivative  Commented=on
  Derivative2 : Derivative  Commented=on
  Divide : Product  Commented=on  Inputs=**/
  From64 : From  Commented=on  GotoTag=w1_sq  TagVisibility=global
  From65 : From  Commented=on  GotoTag=w2_sq  TagVisibility=global
  From66 : From  Commented=on  GotoTag=w3_sq  TagVisibility=global
  From67 : From  Commented=on  GotoTag=w4_sq  TagVisibility=global
  Goto7 : Goto  Commented=on  GotoTag=yd  TagVisibility=global
  PID Controller : simulink/Continuous/PID Controller  Controller=PID  TimeDomain=Continuous-time  SampleTime=-1  IntegratorMethod=Forward Euler  FilterMethod=Forward Euler  Form=Parallel  UseFilter=on  ControllerParametersSource=internal  P=Kp_y  I=Ki_y  D=Kd_y  N=100  InitialConditionSource=internal  InitialConditionForIntegrator=0  InitialConditionForFilter=0  ExternalReset=none  LimitOutput=off  UpperSaturationLimit=inf  LowerSaturationLimit=-inf  LinearizeAsGain=on  AntiWindupMode=none  Kb=1  TrackingMode=off  Kt=1  PParamMin=[]  PParamMax=[]  IParamMin=[]  IParamMax=[]  DParamMin=[]  DParamMax=[]  NParamMin=[]  NParamMax=[]  KbParamMin=[]  KbParamMax=[]  KtParamMin=[]  KtParamMax=[]  POutMin=[]  POutMax=[]  IOutMin=[]  IOutMax=[]  DOutMin=[]  DOutMax=[]  NOutMin=[]  NOutMax=[]  KbOutMin=[]  KbOutMax=[]  KtOutMin=[]  KtOutMax=[]  IntegratorOutMin=[]  IntegratorOutMax=[]  FilterOutMin=[]  FilterOutMax=[]  SumOutMin=[]  SumOutMax=[]  SumI1OutMin=[]  SumI1OutMax=[]  SumI2OutMin=[]  SumI2OutMax=[]  SumI3OutMin=[]  SumI3OutMax=[]  SumDOutMin=[]  SumDOutMax=[]  SaturationOutMin=[]  SaturationOutMax=[]  IntegratorContinuousStateAttributes=''  IntegratorStateMustResolveToSignalObject=off  IntegratorRTWStateStorageClass=Auto  FilterContinuousStateAttributes=''  FilterStateMustResolveToSignalObject=off  FilterRTWStateStorageClass=Auto  DifferentiatorICPrevScaledInput=0  DifferentiatorOutMin=[]  DifferentiatorOutMax=[]
  Sum5 : Sum  Commented=on  Inputs=++++  OutMin=[0.0001]
  Sum7 : Sum  Inputs=-+|
  pitch_TF2 : TransferFcn  Commented=on  Denominator=[tau_p 1]
  Out1 : Outport
  wires:
  [yd] -> Sum7/2, pitch_TF2/1
  From65/1 -> Sum5/2
  From64/1 -> Sum5/1
  From67/1 -> Sum5/4
  Sum5/1 -> Divide/3
  From66/1 -> Sum5/3
  In1/1 -> Sum7/1
  Constant/1 -> Divide/2
  Derivative/1 -> Derivative2/1
  Sum7/1 -> PID Controller/1
  PID Controller/1 -> Out1/1
  pitch_TF2/1 -> Goto7/1

== system all_sliding_mode_z_trajectory_extension_v1/PID/T_phi ==
  phi ref : Inport
  Derivative2 : Derivative
  Gain7 : Gain  Gain=Kp_phi
  Gain8 : Gain  Gain=Ki_phi
  Gain9 : Gain  Gain=Kd_phi
  Integrator10 : Integrator
  Product11 : Product
  Saturation1 : Saturate  UpperLimit=2000  LowerLimit=-2000
  Scope1 : Scope  NumInputPorts=5
  Sine Wave : Sin  Amplitude=disturbance  Frequency=fd  SampleTime=0
  Sum6 : Sum  Inputs=|+++
  Sum7 : Sum  Inputs=|+-+
  b/m10 : Constant  Value=Ixx
  T_phi : Outport
  wires:
  b/m10/1 -> Product11/1
  Derivative2/1 -> Sum6/3
  Gain8/1 -> Integrator10/1
  Gain9/1 -> Derivative2/1
  Gain7/1 -> Sum6/1
  Integrator10/1 -> Sum6/2
  Saturation1/1 -> T_phi/1
  Sum6/1 -> Scope1/2, Product11/2, [w_z_pid]
  phi ref/1 -> Scope1/5, Sum7/1
  Sum7/1 -> Scope1/1, Gain7/1, Gain9/1, Gain8/1
  [phi_actual] -> Scope1/4, Sum7/2
  Product11/1 -> Scope1/3, Saturation1/1
  Sine Wave/1 -> Sum7/3

== system all_sliding_mode_z_trajectory_extension_v1/PID/T_psi ==
  psi ref : Inport
  Derivative2 : Derivative
  Gain7 : Gain  Gain=Kp_z
  Gain8 : Gain  Gain=Ki_z
  Gain9 : Gain  Gain=Kd_z
  Integrator10 : Integrator
  Product11 : Product
  Saturation6 : Saturate  UpperLimit=4000  LowerLimit=-4000
  Scope1 : Scope  NumInputPorts=5
  Sine Wave : Sin  Amplitude=disturbance  Frequency=fd  SampleTime=0
  Sum6 : Sum  Inputs=|+++
  Sum7 : Sum  Inputs=|+-+
  b/m10 : Constant  Value=Ixx
  T_psi : Outport
  wires:
  b/m10/1 -> Product11/1
  Derivative2/1 -> Sum6/3
  Gain8/1 -> Integrator10/1
  Gain9/1 -> Derivative2/1
  Gain7/1 -> Sum6/1
  Integrator10/1 -> Sum6/2
  Saturation6/1 -> T_psi/1
  Sum6/1 -> Product11/2, Scope1/2, [w_z_pid]
  psi ref/1 -> Scope1/5, Sum7/1
  Sum7/1 -> Scope1/1, Gain9/1, Gain7/1, Gain8/1
  [psi_actual] -> Scope1/4, Sum7/2
  Product11/1 -> Scope1/3, Saturation6/1
  Sine Wave/1 -> Sum7/3

== system all_sliding_mode_z_trajectory_extension_v1/PID/T_theta ==
  theta ref : Inport
  Derivative2 : Derivative
  Gain7 : Gain  Gain=Kp_theta
  Gain8 : Gain  Gain=Ki_theta
  Gain9 : Gain  Gain=Kd_theta
  Integrator10 : Integrator
  Product11 : Product
  Saturation1 : Saturate  UpperLimit=2000  LowerLimit=-2000
  Scope1 : Scope  NumInputPorts=5
  Sine Wave : Sin  Amplitude=disturbance  Frequency=fd  SampleTime=0
  Sum6 : Sum  Inputs=|+++
  Sum7 : Sum  Inputs=|+-+
  b/m10 : Constant  Value=Ixx
  T_theta : Outport
  wires:
  Sum6/1 -> Product11/2, Scope1/2, [w_theta_pid]
  b/m10/1 -> Product11/1
  theta ref/1 -> Scope1/5, Sum7/1
  Derivative2/1 -> Sum6/3
  Sum7/1 -> Gain8/1, Gain9/1, Gain7/1, Scope1/1
  Gain8/1 -> Integrator10/1
  Gain9/1 -> Derivative2/1
  Gain7/1 -> Sum6/1
  Integrator10/1 -> Sum6/2
  [theta_actual] -> Scope1/4, Sum7/2
  Product11/1 -> Scope1/3, Saturation1/1
  Saturation1/1 -> T_theta/1
  Sine Wave/1 -> Sum7/3

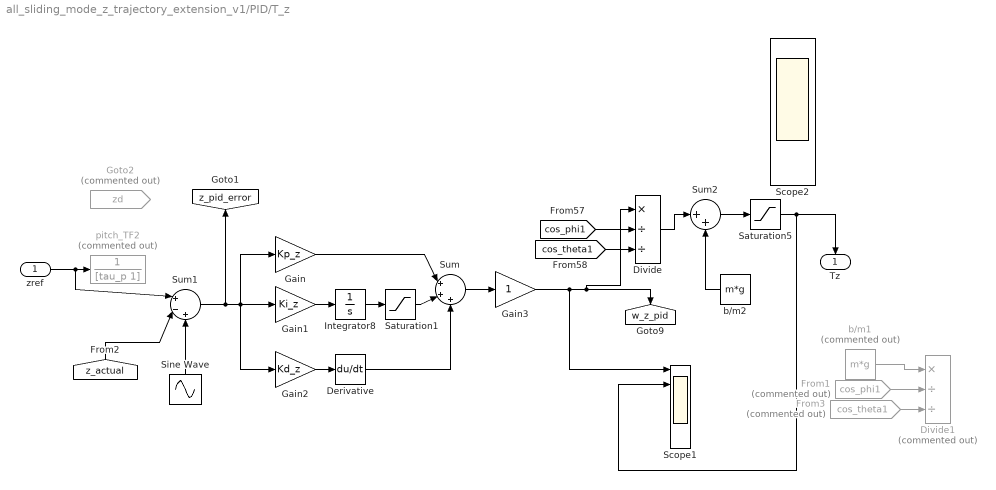
== system all_sliding_mode_z_trajectory_extension_v1/PID/T_z ==
  zref : Inport
  Derivative : Derivative
  Divide : Product  Inputs=*//
  Divide1 : Product  Commented=on  Inputs=*//
  From1 : From  Commented=on  GotoTag=cos_phi1  TagVisibility=global
  From3 : From  Commented=on  GotoTag=cos_theta1  TagVisibility=global
  Gain : Gain  Gain=Kp_z
  Gain1 : Gain  Gain=Ki_z
  Gain2 : Gain  Gain=Kd_z
  Gain3 : Gain
  Goto2 : Goto  Commented=on  GotoTag=zd  TagVisibility=global
  Integrator8 : Integrator
  Saturation1 : Saturate  UpperLimit=10  LowerLimit=-10
  Saturation5 : Saturate  UpperLimit=1000  LowerLimit=0
  Scope1 : Scope  NumInputPorts=6
  Scope2 : Scope  NumInputPorts=4
  Sine Wave : Sin  Amplitude=disturbance * 5  Frequency=fd  SampleTime=0
  Sum : Sum  Inputs=|+++
  Sum1 : Sum  Inputs=|+-+
  Sum2 : Sum  Inputs=|++
  b/m1 : Constant  Commented=on  Value=m*g
  b/m2 : Constant  Value=m*g
  pitch_TF2 : TransferFcn  Commented=on  Denominator=[tau_p 1]
  Tz : Outport
  tag scope: w_z_pid=global, z_pid_error=global
  wires:
  Sum1/1 -> [z_pid_error], Gain1/1, Gain2/1, Gain/1
  Integrator8/1 -> Saturation1/1
  [z_actual] -> Sum1/2
  Gain1/1 -> Integrator8/1
  Gain/1 -> Sum/1
  Gain2/1 -> Derivative/1
  Derivative/1 -> Sum/3
  Sum/1 -> Gain3/1
  Gain3/1 -> Divide/1, [w_z_pid], Scope1/1
  Saturation5/1 -> Tz/1, Scope1/2
  [cos_theta1] -> Divide/3
  [cos_phi1] -> Divide/2
  Sum2/1 -> Saturation5/1
  Saturation1/1 -> Sum/2
  Sine Wave/1 -> Sum1/3
  zref/1 -> Sum1/1, pitch_TF2/1
  b/m1/1 -> Divide1/1
  From3/1 -> Divide1/3
  From1/1 -> Divide1/2
  Divide/1 -> Sum2/1
  b/m2/1 -> Sum2/2

== system all_sliding_mode_z_trajectory_extension_v1/SM Controller/Subsystem10 ==
  note: zd_dot
  Divide6 : Product  Inputs=**
  Sum6 : Sum  Inputs=+-+
  Sum7 : Sum  Inputs=+-
  m*g4 : Constant  Value=a3
  s3 : Outport
  wires:
  [zd_dot] -> Sum6/2
  Sum7/1 -> Divide6/2
  m*g4/1 -> Divide6/1
  [z_dot_actual] -> Sum6/1
  [z_actual] -> Sum7/1
  Divide6/1 -> Sum6/3
  Sum6/1 -> s3/1
  [zd] -> Sum7/2

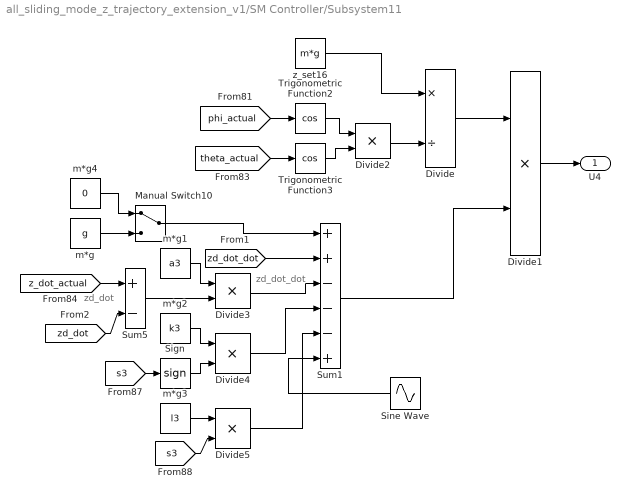
== system all_sliding_mode_z_trajectory_extension_v1/SM Controller/Subsystem11 ==
  note: zd_dot
  note: zd_dot_dot
  Divide : Product  Inputs=*/
  Divide{1..5} (5 alike) : Product  Inputs=**
  Manual Switch10 : ManualSwitch
  Sign : Signum
  Sine Wave : Sin  Amplitude=disturbance*5  Frequency=fd  SampleTime=0
  Sum1 : Sum  Inputs=++---+
  Sum5 : Sum  Inputs=+-
  Trigonometric Function2 : Trigonometry  Operator=cos
  Trigonometric Function3 : Trigonometry  Operator=cos
  m*g : Constant  Value=g
  m*g1 : Constant  Value=a3
  m*g2 : Constant  Value=k3
  m*g3 : Constant  Value=l3
  m*g4 : Constant  Value=0
  z_set16 : Constant  Value=m*g
  U4 : Outport
  wires:
  [zd_dot_dot] -> Sum1/2
  [zd_dot] -> Sum5/2
  Sign/1 -> Divide4/2
  Divide4/1 -> Sum1/4
  Divide1/1 -> U4/1
  m*g1/1 -> Divide3/1
  m*g2/1 -> Divide4/1
  Trigonometric Function2/1 -> Divide2/1
  Divide3/1 -> Sum1/3
  [z_dot_actual] -> Sum5/1
  Trigonometric Function3/1 -> Divide2/2
  Sum5/1 -> Divide3/2
  [s3] -> Divide5/2
  Sum1/1 -> Divide1/2
  [s3] -> Sign/1
  Divide/1 -> Divide1/1
  Divide5/1 -> Sum1/5
  m*g3/1 -> Divide5/1
  Divide2/1 -> Divide/2
  [phi_actual] -> Trigonometric Function2/1
  [theta_actual] -> Trigonometric Function3/1
  z_set16/1 -> Divide/1
  m*g/1 -> Manual Switch10/2
  m*g4/1 -> Manual Switch10/1
  Manual Switch10/1 -> Sum1/1
  Sine Wave/1 -> Sum1/6

== system all_sliding_mode_z_trajectory_extension_v1/SM Controller/Subsystem12 ==
  note: xd_dot
  note: xd_dot
  Divide6 : Product  Inputs=**
  Sum6 : Sum  Inputs=+-+
  Sum7 : Sum  Inputs=+-
  m*g4 : Constant  Value=a1
  s1 : Outport
  wires:
  Sum6/1 -> s1/1
  Divide6/1 -> Sum6/3
  [x_actual] -> Sum7/1
  [xactual_dot] -> Sum6/1
  m*g4/1 -> Divide6/1
  Sum7/1 -> Divide6/2
  [xd_dot] -> Sum6/2
  [xd] -> Sum7/2

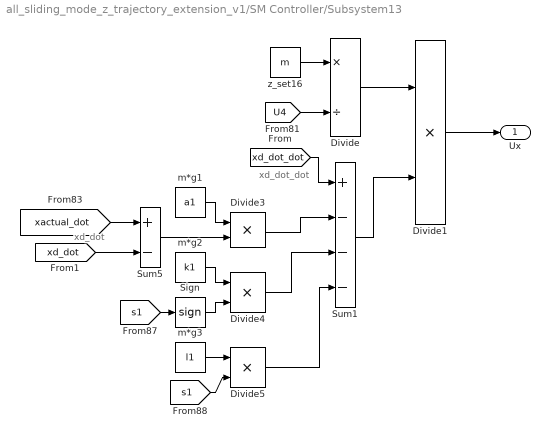
== system all_sliding_mode_z_trajectory_extension_v1/SM Controller/Subsystem13 ==
  note: xd_dot
  note: xd_dot_dot
  Divide : Product  Inputs=*/
  Divide{1,3..5} (4 alike) : Product  Inputs=**
  Sign : Signum
  Sum1 : Sum  Inputs=+---
  Sum5 : Sum  Inputs=+-
  m*g1 : Constant  Value=a1
  m*g2 : Constant  Value=k1
  m*g3 : Constant  Value=l1
  z_set16 : Constant  Value=m
  Ux : Outport
  wires:
  m*g2/1 -> Divide4/1
  [xactual_dot] -> Sum5/1
  [xd_dot] -> Sum5/2
  [xd_dot_dot] -> Sum1/1
  Sum1/1 -> Divide1/2
  m*g3/1 -> Divide5/1
  z_set16/1 -> Divide/1
  Sign/1 -> Divide4/2
  Divide5/1 -> Sum1/4
  Divide/1 -> Divide1/1
  Divide1/1 -> Ux/1
  Sum5/1 -> Divide3/2
  [s1] -> Divide5/2
  [s1] -> Sign/1
  [U4] -> Divide/2
  m*g1/1 -> Divide3/1
  Divide3/1 -> Sum1/2
  Divide4/1 -> Sum1/3

== system all_sliding_mode_z_trajectory_extension_v1/SM Controller/Subsystem14 ==
  note: yd_dot_dot
  note: yd_dot
  Divide : Product  Inputs=*/
  Divide{1,3..5} (4 alike) : Product  Inputs=**
  Sign : Signum
  Sum1 : Sum  Inputs=+---
  Sum5 : Sum  Inputs=+-
  m*g1 : Constant  Value=a2
  m*g2 : Constant  Value=k2
  m*g3 : Constant  Value=l2
  z_set16 : Constant  Value=m
  Uy : Outport
  wires:
  Divide3/1 -> Sum1/2
  m*g1/1 -> Divide3/1
  [U4] -> Divide/2
  [s2] -> Sign/1
  [s2] -> Divide5/2
  Sum5/1 -> Divide3/2
  Divide1/1 -> Uy/1
  Divide/1 -> Divide1/1
  Divide5/1 -> Sum1/4
  Sign/1 -> Divide4/2
  z_set16/1 -> Divide/1
  m*g3/1 -> Divide5/1
  Sum1/1 -> Divide1/2
  [yd_dot_dot] -> Sum1/1
  [yd_dot] -> Sum5/2
  [yactual_dot] -> Sum5/1
  m*g2/1 -> Divide4/1
  Divide4/1 -> Sum1/3

== system all_sliding_mode_z_trajectory_extension_v1/SM Controller/Subsystem15 ==
  note: yd_dot
  Divide6 : Product  Inputs=**
  Sum6 : Sum  Inputs=+-+
  Sum7 : Sum  Inputs=+-
  m*g4 : Constant  Value=a2
  s2 : Outport
  wires:
  [yd_dot] -> Sum6/2
  Sum7/1 -> Divide6/2
  m*g4/1 -> Divide6/1
  [yactual_dot] -> Sum6/1
  [y_actual] -> Sum7/1
  Divide6/1 -> Sum6/3
  Sum6/1 -> s2/1
  [yd] -> Sum7/2

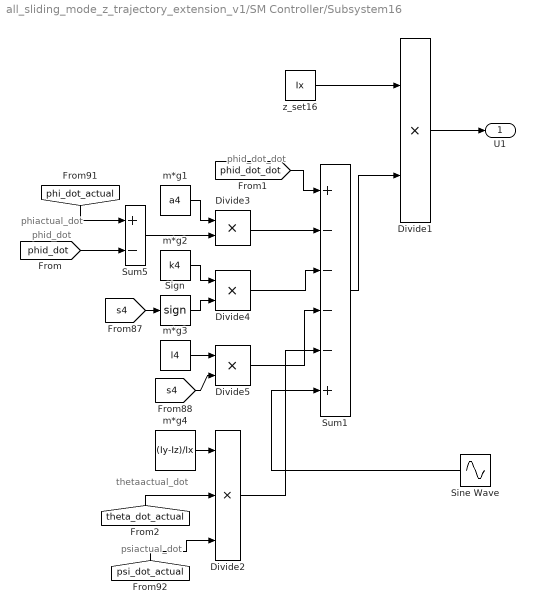
== system all_sliding_mode_z_trajectory_extension_v1/SM Controller/Subsystem16 ==
  note: psiactual_dot
  note: thetaactual_dot
  note: phid_dot_dot
  note: phid_dot
  note: phiactual_dot
  Divide{1,3..5} (4 alike) : Product  Inputs=**
  Divide2 : Product  Inputs=***
  Sign : Signum
  Sine Wave : Sin  Amplitude=disturbance  Frequency=fd  SampleTime=0
  Sum1 : Sum  Inputs=+----+
  Sum5 : Sum  Inputs=+-
  m*g1 : Constant  Value=a4
  m*g2 : Constant  Value=k4
  m*g3 : Constant  Value=l4
  m*g4 : Constant  Value=(Iy-Iz)/Ix
  z_set16 : Constant  Value=Ix
  U1 : Outport
  wires:
  Divide4/1 -> Sum1/3
  Divide3/1 -> Sum1/2
  m*g1/1 -> Divide3/1
  [s4] -> Sign/1
  [s4] -> Divide5/2
  Sum5/1 -> Divide3/2
  Divide1/1 -> U1/1
  z_set16/1 -> Divide1/1
  Divide5/1 -> Sum1/4
  Sign/1 -> Divide4/2
  m*g3/1 -> Divide5/1
  Sum1/1 -> Divide1/2
  [phid_dot_dot] -> Sum1/1
  [phid_dot] -> Sum5/2
  [phi_dot_actual] -> Sum5/1
  m*g2/1 -> Divide4/1
  Divide2/1 -> Sum1/5
  [theta_dot_actual] -> Divide2/2
  m*g4/1 -> Divide2/1
  [psi_dot_actual] -> Divide2/3
  Sine Wave/1 -> Sum1/6

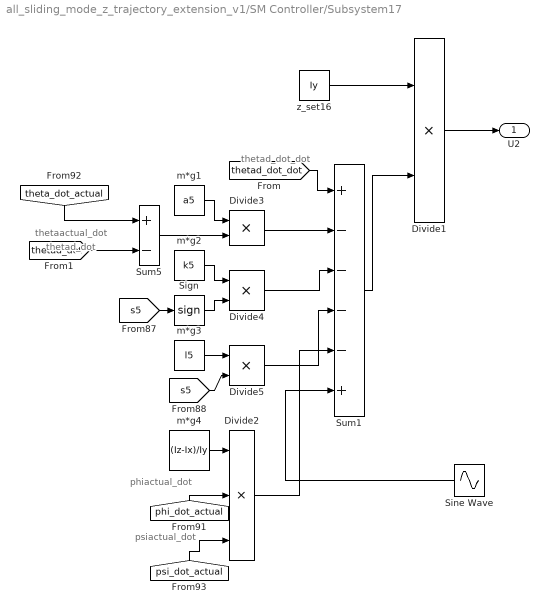
== system all_sliding_mode_z_trajectory_extension_v1/SM Controller/Subsystem17 ==
  note: thetaactual_dot
  note: thetad_dot
  note: thetad_dot_dot
  note: phiactual_dot
  note: psiactual_dot
  Divide{1,3..5} (4 alike) : Product  Inputs=**
  Divide2 : Product  Inputs=***
  Sign : Signum
  Sine Wave : Sin  Amplitude=disturbance  Frequency=fd  SampleTime=0
  Sum1 : Sum  Inputs=+----+
  Sum5 : Sum  Inputs=+-
  m*g1 : Constant  Value=a5
  m*g2 : Constant  Value=k5
  m*g3 : Constant  Value=l5
  m*g4 : Constant  Value=(Iz-Ix)/Iy
  z_set16 : Constant  Value=Iy
  U2 : Outport
  wires:
  [psi_dot_actual] -> Divide2/3
  m*g4/1 -> Divide2/1
  [phi_dot_actual] -> Divide2/2
  Divide2/1 -> Sum1/5
  m*g2/1 -> Divide4/1
  [theta_dot_actual] -> Sum5/1
  [thetad_dot] -> Sum5/2
  [thetad_dot_dot] -> Sum1/1
  Sum1/1 -> Divide1/2
  m*g3/1 -> Divide5/1
  Sign/1 -> Divide4/2
  Divide5/1 -> Sum1/4
  z_set16/1 -> Divide1/1
  Divide1/1 -> U2/1
  Sum5/1 -> Divide3/2
  [s5] -> Divide5/2
  [s5] -> Sign/1
  m*g1/1 -> Divide3/1
  Divide3/1 -> Sum1/2
  Divide4/1 -> Sum1/3
  Sine Wave/1 -> Sum1/6

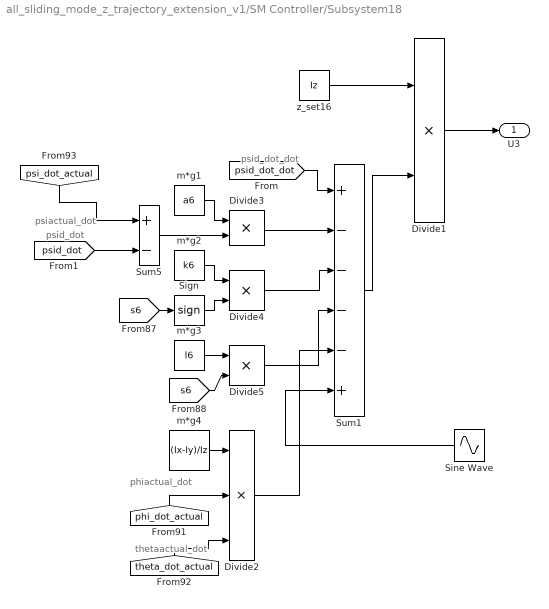
== system all_sliding_mode_z_trajectory_extension_v1/SM Controller/Subsystem18 ==
  note: thetaactual_dot
  note: phiactual_dot
  note: psid_dot_dot
  note: psid_dot
  note: psiactual_dot
  Divide{1,3..5} (4 alike) : Product  Inputs=**
  Divide2 : Product  Inputs=***
  Sign : Signum
  Sine Wave : Sin  Amplitude=disturbance  Frequency=fd  SampleTime=0
  Sum1 : Sum  Inputs=+----+
  Sum5 : Sum  Inputs=+-
  m*g1 : Constant  Value=a6
  m*g2 : Constant  Value=k6
  m*g3 : Constant  Value=l6
  m*g4 : Constant  Value=(Ix-Iy)/Iz
  z_set16 : Constant  Value=Iz
  U3 : Outport
  wires:
  Divide4/1 -> Sum1/3
  Divide3/1 -> Sum1/2
  m*g1/1 -> Divide3/1
  [s6] -> Sign/1
  [s6] -> Divide5/2
  Sum5/1 -> Divide3/2
  Divide1/1 -> U3/1
  z_set16/1 -> Divide1/1
  Divide5/1 -> Sum1/4
  Sign/1 -> Divide4/2
  m*g3/1 -> Divide5/1
  Sum1/1 -> Divide1/2
  [psid_dot_dot] -> Sum1/1
  [psid_dot] -> Sum5/2
  [psi_dot_actual] -> Sum5/1
  m*g2/1 -> Divide4/1
  Divide2/1 -> Sum1/5
  [phi_dot_actual] -> Divide2/2
  m*g4/1 -> Divide2/1
  [theta_dot_actual] -> Divide2/3
  Sine Wave/1 -> Sum1/6

== system all_sliding_mode_z_trajectory_extension_v1/SM Controller/Subsystem19 ==
  note: yd_dot
  Divide6 : Product  Inputs=**
  Sum6 : Sum  Inputs=+-+
  Sum7 : Sum  Inputs=+-
  m*g4 : Constant  Value=a4
  s4 : Outport
  wires:
  Sum6/1 -> s4/1
  Divide6/1 -> Sum6/3
  [phi_actual] -> Sum7/1
  [phi_dot_actual] -> Sum6/1
  m*g4/1 -> Divide6/1
  Sum7/1 -> Divide6/2
  [phi_set] -> Sum7/2
  [phid_dot] -> Sum6/2

== system all_sliding_mode_z_trajectory_extension_v1/SM Controller/Subsystem20 ==
  note: yd_dot
  Divide6 : Product  Inputs=**
  Sum6 : Sum  Inputs=+-+
  Sum7 : Sum  Inputs=+-
  m*g4 : Constant  Value=a5
  s5 : Outport
  wires:
  [thetad_dot] -> Sum6/2
  [theta_set] -> Sum7/2
  Sum7/1 -> Divide6/2
  m*g4/1 -> Divide6/1
  [theta_dot_actual] -> Sum6/1
  [theta_actual] -> Sum7/1
  Divide6/1 -> Sum6/3
  Sum6/1 -> s5/1

== system all_sliding_mode_z_trajectory_extension_v1/SM Controller/Subsystem21 ==
  note: yd_dot
  Divide6 : Product  Inputs=**
  Sum6 : Sum  Inputs=+-+
  Sum7 : Sum  Inputs=+-
  m*g4 : Constant  Value=a6
  pitch_TF : TransferFcn  Commented=on  Denominator=[tau_att 1]
  z_set3 : Constant  Value=psi_ref
  s6 : Outport
  wires:
  Sum6/1 -> s6/1
  Divide6/1 -> Sum6/3
  [psi_actual] -> Sum7/1
  [psi_dot_actual] -> Sum6/1
  m*g4/1 -> Divide6/1
  Sum7/1 -> Divide6/2
  z_set3/1 -> Sum7/2, pitch_TF/1
  [psid_dot] -> Sum6/2
